simulink model "Assignment1_2020a"  (R2020a)
settings: Solver=FixedStepAuto  StartTime=0.0  StopTime=30  FixedStep=1e-3  RelTol=1e-3  EnableMultiTasking=on
undefined symbols (not defined in the file): A0, A1, D0, D1, D10, D11, D12, D13, D2, D3, D4, D5, D6, D7, D8, D9, PTA0, PTA1, PTA2, PTB2, PTB23, PTB3, PTB9, PTC16, PTC17, PTC2, PTC3, PTC4, PTD0, PTD1, PTD2, PTD3
libraries: frdmk64flib x23, etargetslib x2, dspstat3 x1
settings Model: ExtModeTrigDuration=5  Creator=raymo  LastModifiedBy=raymo
settings OptimizationCC: EnhancedBackFolding=on  PassReuseOutputArgsAs=Individual arguments  ZeroExternalMemoryAtStartup=off  ZeroInternalMemoryAtStartup=off  MaxStackSize=64  OptimizeBlockOrder=speed  DifferentSizesBufferReuse=on  OptimizationCustomize=off  EfficientTunableParamExpr=on
settings DebuggingCC: ParameterTunabilityLossMsg=error
settings HardwareCC: ProdBitPerPointer=32  ProdBitPerSizeT=32  ProdBitPerPtrDiffT=32  ProdLargestAtomicInteger=Long  ProdLargestAtomicFloat=Double  ProdWordSize=32  ProdHWDeviceType=ARM Compatible->ARM Cortex
settings SFSimCC: MATLABDynamicMemAlloc=off
settings RTWCC: SystemTargetFile=ert.tlc  HardwareBoard=NXP FRDM-K64F  TemplateMakefile=ert_default_tmf  Toolchain=GNU Tools for ARM Embedded Processors
settings CodeAppCC: ForceParamTrailComments=on  IgnoreCustomStorageClasses=off  OperatorAnnotations=on  SimulinkDataObjDesc=on  SFDataObjDesc=on  InsertBlockDesc=on

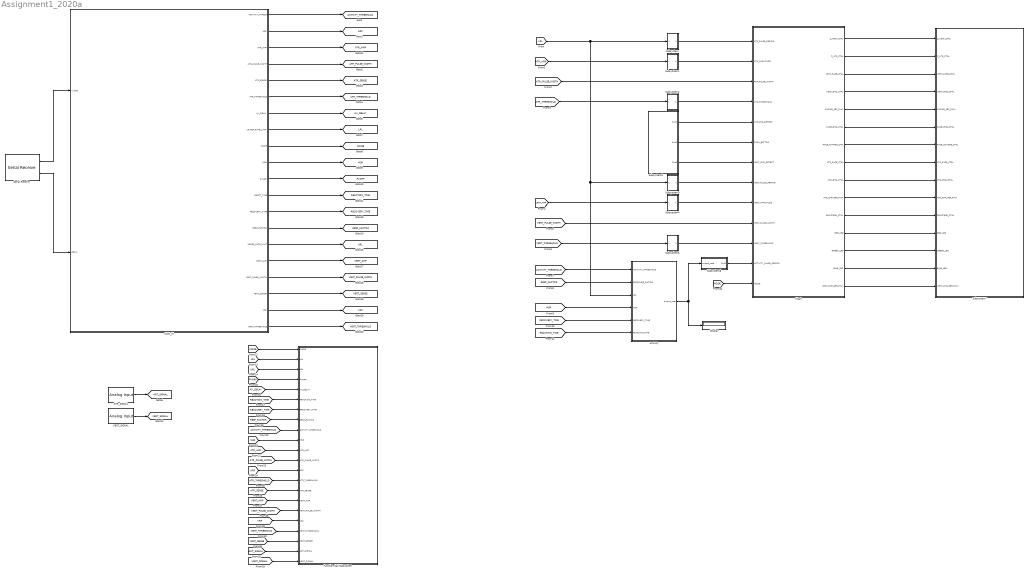
== system Assignment1_2020a ==
  ATR_SIGNAL : frdmk64flib/Analog Input  Whichpin=PTB2 (A0)  SampleTime=-1
  Activity : Subsystem
  COM_IN : Stateflow chart  TreatAsAtomicUnit=on
  Chart : Stateflow chart  TreatAsAtomicUnit=on
      settings: PortSchema="{\"entries\":[{\"content\":{\"sides\":[{\"content\":{\"connectorIds\":[\"In1\",\"In2\",\"In3\",\"In4\",\"In5\",\"In6\",\"In9\",\"In7\",\"In8\",\"In10\",\"In11\",\"In12\",\"In13\"]},\"type\":\"ConnectorPlacement.EquallySpacedRectSide\",\"uuid\":\"1d074b9c-7cc8-4198-85a6-5618993573f0\"},{\"content\":{\"connectorIds\":[\"Out1\",\"Out2\",\"Out3\",\"Out4\",\"Out5\",\"Out6\",\"Out7\",\"Out8\",\"Out9\",\"Out10\",\"Out11\",\"Out12\",\"Out13\",\"Out14\",\"Out15\"],\"side\":\"RIGHT\"},\"type\":\"ConnectorPlacement.EquallySpacedRectSide\",\"uuid\":\"14c2042e-8be8-4cb1-bcfb-7c1019a33e21\"},{\"content\":{\"connectorIds\":[],\"side\":\"TOP\"},\"type\":\"ConnectorPlacement.EquallySpacedRectSide\",\"uuid\":\"e4fcd7b9-cecf-490a-a51f-afb907c3ace7\"}]},\"type\":\"ConnectorPlacement.EquallySpacedConnector\",\"uuid\":\"e4f7c1e4-ab35-4f24-879f-75d9e4e0e882\"}],\"packageUris\":[\"http://schema.mathworks.com/mf0/Connector/19700101\"],\"version\":\"1.0\"}"
  Display : Display
  Function-Call Subsystem : Subsystem  TreatAsAtomicUnit=on
  Serial Receive : frdmk64flib/Serial Receive  SCIModule=0  Baudrate=uint32(9600)  Parity=None  StopBits=1  HardwareFlowControl=None  ByteOrder=LittleEndian  DataType=uint8  DataLength=11  BlockingMode=off  OutputStatus=on  SampleTime=-1
  Subsystem : Subsystem
  Subsystem1 : Subsystem
  Subsystem2 : Subsystem
  Subsystem3 : Subsystem
  Subsystem4 : Subsystem
  Subsystem5 : Subsystem
  Subsystem6 : Subsystem
  Subsystem7 : Subsystem
  Subsystem8 : Subsystem
  VENT_SIGNAL : frdmk64flib/Analog Input  Whichpin=PTB3 (A1)  SampleTime=-1
  tag scope: ACTIVITY_THRESHOLD=global, ARP=global, ART_SIGNAL=global, ATR_AMP=global, ATR_PULSE_WIDTH=global, ATR_SENSE=global, ATR_THRESHOLD=global, AV_DELAY=global, LRL=global, MODE=global, MSR=global, PVARP=global, REACTION_TIME=global, RECOVERY_TIME=global, RESP_FACTOR=global, URL=global, VENT_AMP=global, VENT_PULSE_WIDTH=global, VENT_SENSE=global, VENT_SIGNAL=global, VENT_THRESHOLD=global, VRP=global
  wires:
  [ATR_PULSE_WIDTH] -> Chart/3(ATR_PULSE_WIDTH)
  Subsystem/1(Out1) -> Chart/1(ATR_PULSE_PERIOD)
  [ATR_AMP] -> Subsystem1/1(In1)
  Subsystem1/1(Out1) -> Chart/2(ATR_AMPLITUDE)
  [ATR_THRESHOLD] -> Subsystem2/1(In1)
  Subsystem2/1(Out1) -> Chart/4(ATR_THRESHOLD)
  Subsystem3/1(Out1) -> Chart/7(VENT_PULSE_PERIOD)
  [LRL] -> Subsystem3/1(In1), Activity/3(LRL), Subsystem/1(In1)
  [VENT_AMP] -> Subsystem4/1(In1)
  Subsystem4/1(Out1) -> Chart/8(VENT_AMPLITUDE)
  [VENT_THRESHOLD] -> Subsystem5/1(In1)
  Subsystem5/1(Out1) -> Chart/11(VENT_THRESHOLD)
  Subsystem6/1(Out1) -> Chart/5(ATR_CMP_DETECT)
  Subsystem6/2(Out2) -> Chart/6(PUSH_BUTTON)
  Subsystem6/3(Out3) -> Chart/9(VENT_CMP_DETECT)
  Chart/1(Z_VENT_CTRL) -> Subsystem7/1(Z_VENT_CTRL)
  Chart/2(Z_ATR_CTRL) -> Subsystem7/2(Z_ATR_CTRL)
  Chart/3(VENT_PACE_CTRL) -> Subsystem7/3(VENT_PACE_CTRL)
  Chart/4(VENT_GND_CTRL) -> Subsystem7/4(VENT_GND_CTRL)
  Chart/5(PACING_REF_PWM) -> Subsystem7/5(PACING_REF_PWM)
  Chart/6(PACE_GND_CTRL) -> Subsystem7/6(PACE_GND_CTRL)
  Chart/7(PACE_CHARGE_CTRL) -> Subsystem7/7(PACE_CHARGE_CTRL)
  Chart/8(ATR_PACE_CTRL) -> Subsystem7/8(ATR_PACE_CTRL)
  Chart/9(ATR_GND_CTRL) -> Subsystem7/9(ATR_GND_CTRL)
  Chart/10(ATR_CMP_REF_PWM) -> Subsystem7/10(ATR_CMP_REF_PWM)
  Chart/11(FRONTEND_CTRL) -> Subsystem7/11(FRONTEND_CTRL)
  Chart/12(RED_LED) -> Subsystem7/12(RED_LED)
  Chart/13(GREEN_LED) -> Subsystem7/13(GREEN_LED)
  Chart/15(VENT_CMP_REF_PWM) -> Subsystem7/15(VENT_CMP_REF_PWM)
  Activity/1(output_rate) -> Display/1, Subsystem8/1(output_rate)
  Subsystem8/1(Out1) -> Chart/12(ACTIVITY_PULSE_PERIOD)
  Chart/14(BLUE_LED) -> Subsystem7/14(BLUE_LED)
  Serial Receive/1 -> COM_IN/1(rxdata)
  Serial Receive/2 -> COM_IN/2(status)
  COM_IN/1(ACTIVITY_THRESH) -> [ACTIVITY_THRESHOLD]
  COM_IN/2(ARP) -> [ARP]
  COM_IN/3(ATR_AMP) -> [ATR_AMP]
  COM_IN/4(ATR_PULSE_WIDTH) -> [ATR_PULSE_WIDTH]
  COM_IN/5(ATR_SENSE) -> [ATR_SENSE]
  COM_IN/8(LOWER_RATE_LIMIT) -> [LRL]
  COM_IN/6(ATR_THRESHOLD) -> [ATR_THRESHOLD]
  COM_IN/7(AV_DELAY) -> [AV_DELAY]
  COM_IN/9(MODE) -> [MODE]
  COM_IN/10(MSR) -> [MSR]
  COM_IN/11(PVARP) -> [PVARP]
  COM_IN/13(RECOVERY_TIME) -> [RECOVERY_TIME]
  COM_IN/12(REACT_TIME) -> [REACTION_TIME]
  COM_IN/16(VENT_AMP) -> [VENT_AMP]
  COM_IN/14(RESP_FACTOR) -> [RESP_FACTOR]
  COM_IN/15(UPPER_RATE_LIMIT) -> [URL]
  COM_IN/18(VENT_SENSE) -> [VENT_SENSE]
  COM_IN/17(VENT_PULSE_WIDTH) -> [VENT_PULSE_WIDTH]
  COM_IN/20(VENT_THRESHOLD) -> [VENT_THRESHOLD]
  COM_IN/19(VRP) -> [VRP]
  [ACTIVITY_THRESHOLD] -> Activity/1(ACTIVITY_THRESHOLD)
  [RESP_FACTOR] -> Activity/2(RESPONSE_FACTOR)
  [MSR] -> Activity/4(MSR)
  [RECOVERY_TIME] -> Activity/5(RECOVERY_TIME)
  [REACTION_TIME] -> Activity/6(REACTION_TIME)
  [MODE] -> Function-Call Subsystem/1(MODE)
  [LRL] -> Function-Call Subsystem/2(LRL)
  [URL] -> Function-Call Subsystem/3(URL)
  [AV_DELAY] -> Function-Call Subsystem/5(AV_DELAY)
  [PVARP] -> Function-Call Subsystem/4(PVARP)
  [REACTION_TIME] -> Function-Call Subsystem/6(REACTION_TIME)
  [RESP_FACTOR] -> Function-Call Subsystem/8(RESP_FACTOR)
  [RECOVERY_TIME] -> Function-Call Subsystem/7(RECOVERY_TIME)
  [ACTIVITY_THRESHOLD] -> Function-Call Subsystem/9(ACTIVITY_TRESHOLD)
  [ATR_AMP] -> Function-Call Subsystem/11(ATR_AMP)
  [MSR] -> Function-Call Subsystem/10(MSR)
  [ATR_PULSE_WIDTH] -> Function-Call Subsystem/12(ATR_PULSE_WIDTH)
  [ATR_THRESHOLD] -> Function-Call Subsystem/14(ATR_THRESHOLD)
  [ARP] -> Function-Call Subsystem/13(ARP)
  [ATR_SENSE] -> Function-Call Subsystem/15(ATR_SENSE)
  [VENT_PULSE_WIDTH] -> Function-Call Subsystem/17(VENT_PULSE_WIDTH)
  [VENT_AMP] -> Function-Call Subsystem/16(VENT_AMP)
  [VRP] -> Function-Call Subsystem/18(VRP)
  [VENT_SIGNAL] -> Function-Call Subsystem/22(VENT_SIGNAL)
  [VENT_THRESHOLD] -> Function-Call Subsystem/19(VENT_THRESHOLD)
  [ART_SIGNAL] -> Function-Call Subsystem/21(ART_SIGNAL)
  [VENT_SENSE] -> Function-Call Subsystem/20(VENT_SENSE)
  ATR_SIGNAL/1 -> [ART_SIGNAL]
  VENT_SIGNAL/1 -> [VENT_SIGNAL]
  [VENT_PULSE_WIDTH] -> Chart/10(VENT_PULSE_WIDTH)
  [MODE] -> Chart/13(MODE)

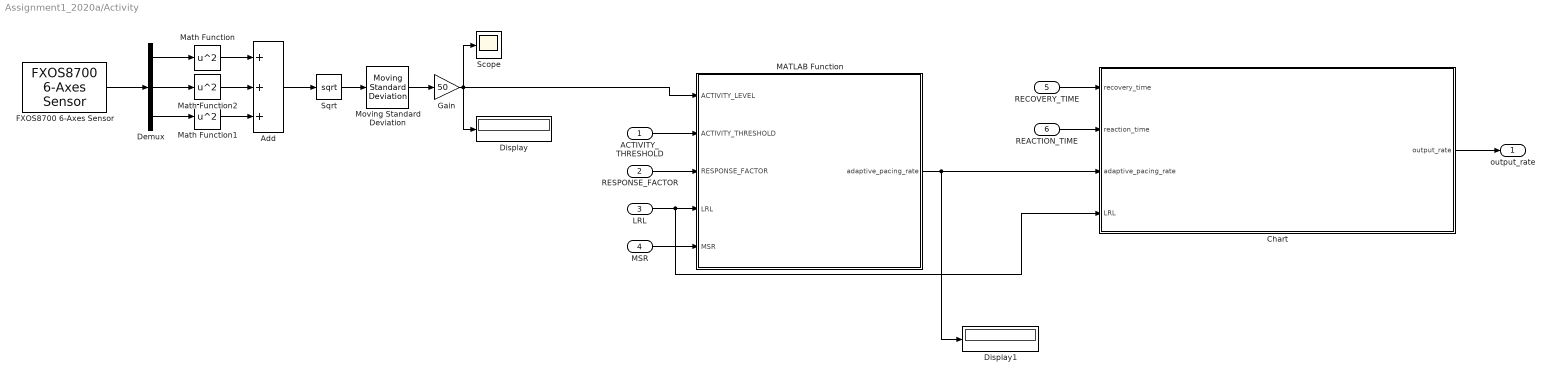
== system Assignment1_2020a/Activity ==
  ACTIVITY_THRESHOLD : Inport
  RESPONSE_FACTOR : Inport  Port=2
  LRL : Inport  Port=3
  MSR : Inport  Port=4
  RECOVERY_TIME : Inport  Port=5
  REACTION_TIME : Inport  Port=6
  Add : Sum  Inputs=+++
  Chart : Stateflow chart  TreatAsAtomicUnit=on
  Demux : Demux  Outputs=3
  Display : Display
  Display1 : Display
  FXOS8700 6-Axes Sensor : frdmk64flib/FXOS8700 6-Axes Sensor  Activesensor=Accelerometer only  ODR=800Hz  HybridODR=400Hz  Accelfullrange=-4g to +4g  SampleTime=-1
  Gain : Gain  Gain=50
  MATLAB Function : MATLAB Function  TreatAsAtomicUnit=on
  Math Function : Math  Operator=square  SaturateOnIntegerOverflow=on
  Math Function1 : Math  Operator=square  SaturateOnIntegerOverflow=on
  Math Function2 : Math  Operator=square  SaturateOnIntegerOverflow=on
  Moving Standard Deviation : dspstat3/Moving Standard Deviation  Method=Sliding window  ForgettingFactorPort=off  SpecifyWindowLength=on  WindowLength=4  ForgettingFactor=0.9  SimulateUsing=Interpreted execution
      settings: SourceProductBaseCode=DS
  Scope : Scope
  Sqrt : Sqrt  SaturateOnIntegerOverflow=on
  output_rate : Outport
  wires:
  FXOS8700 6-Axes Sensor/1 -> Demux/1
  Demux/3 -> Math Function1/1
  Demux/2 -> Math Function2/1
  Demux/1 -> Math Function/1
  Math Function/1 -> Add/1
  Math Function2/1 -> Add/2
  Math Function1/1 -> Add/3
  Add/1 -> Sqrt/1
  Sqrt/1 -> Moving Standard Deviation/1
  Moving Standard Deviation/1 -> Gain/1
  Gain/1 -> Display/1, MATLAB Function/1(ACTIVITY_LEVEL), Scope/1
  ACTIVITY_THRESHOLD/1 -> MATLAB Function/2(ACTIVITY_THRESHOLD)
  RESPONSE_FACTOR/1 -> MATLAB Function/3(RESPONSE_FACTOR)
  LRL/1 -> Chart/4(LRL), MATLAB Function/4(LRL)
  MSR/1 -> MATLAB Function/5(MSR)
  MATLAB Function/1(adaptive_pacing_rate) -> Display1/1, Chart/3(adaptive_pacing_rate)
  RECOVERY_TIME/1 -> Chart/1(recovery_time)
  REACTION_TIME/1 -> Chart/2(reaction_time)
  Chart/1(output_rate) -> output_rate/1

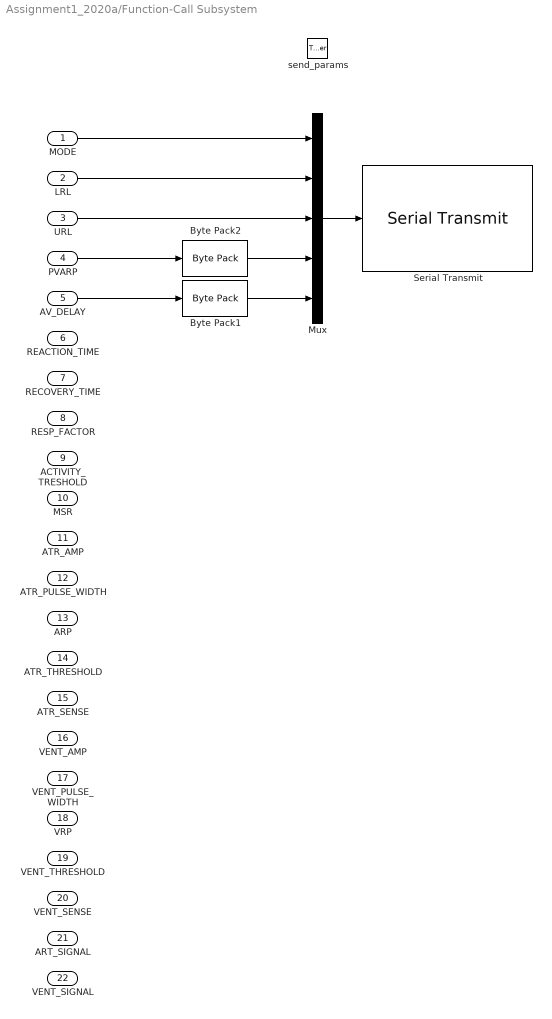
== system Assignment1_2020a/Function-Call Subsystem ==
  MODE : Inport  OutDataTypeStr=uint8
  LRL : Inport  Port=2  OutDataTypeStr=uint8
  URL : Inport  Port=3  OutDataTypeStr=uint8
  PVARP : Inport  Port=4  OutDataTypeStr=single
  AV_DELAY : Inport  Port=5  OutDataTypeStr=uint16
  REACTION_TIME : Inport  Port=6  OutDataTypeStr=uint16
  RECOVERY_TIME : Inport  Port=7  OutDataTypeStr=uint8
  RESP_FACTOR : Inport  Port=8  OutDataTypeStr=uint8
  ACTIVITY_TRESHOLD : Inport  Port=9  OutDataTypeStr=uint8
  MSR : Inport  Port=10  OutDataTypeStr=single
  ATR_AMP : Inport  Port=11  OutDataTypeStr=uint16
  ATR_PULSE_WIDTH : Inport  Port=12  OutDataTypeStr=uint16
  ARP : Inport  Port=13  OutDataTypeStr=uint8
  ATR_THRESHOLD : Inport  Port=14  OutDataTypeStr=uint8
  ATR_SENSE : Inport  Port=15  OutDataTypeStr=uint8
  VENT_AMP : Inport  Port=16  OutDataTypeStr=single
  VENT_PULSE_WIDTH : Inport  Port=17  OutDataTypeStr=uint16
  VRP : Inport  Port=18  OutDataTypeStr=uint16
  VENT_THRESHOLD : Inport  Port=19  OutDataTypeStr=uint8
  VENT_SENSE : Inport  Port=20  OutDataTypeStr=uint8
  ART_SIGNAL : Inport  Port=21  OutDataTypeStr=uint8
  VENT_SIGNAL : Inport  Port=22  OutDataTypeStr=single
  send_params : TriggerPort  TriggerType=function-call  IsSimulinkFunction=on  FunctionName=send_params  VariantControl=Variant
  Byte Pack1 : etargetslib/Byte Pack  datatypes={'uint16'}  byteAlign=1
  Byte Pack2 : etargetslib/Byte Pack  datatypes={'single'}  byteAlign=1
  Mux : Mux  Inputs=5
  Serial Transmit : frdmk64flib/Serial Transmit  SCIModule=0  Baudrate=uint32(9600)  Parity=None  StopBits=1  HardwareFlowControl=None  ByteOrder=LittleEndian  BlockingMode=on  OutputStatus=off
  wires:
  LRL/1 -> Mux/2
  AV_DELAY/1 -> Byte Pack1/1
  Mux/1 -> Serial Transmit/1
  PVARP/1 -> Byte Pack2/1
  Byte Pack1/1 -> Mux/5
  URL/1 -> Mux/3
  MODE/1 -> Mux/1
  Byte Pack2/1 -> Mux/4

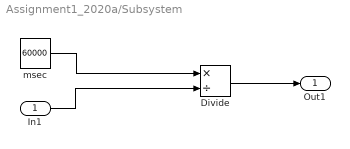
== system Assignment1_2020a/Subsystem ==
  In1 : Inport
  Divide : Product  Inputs=*/
  msec : Constant  Value=60000
  Out1 : Outport
  wires:
  Divide/1 -> Out1/1
  msec/1 -> Divide/1
  In1/1 -> Divide/2

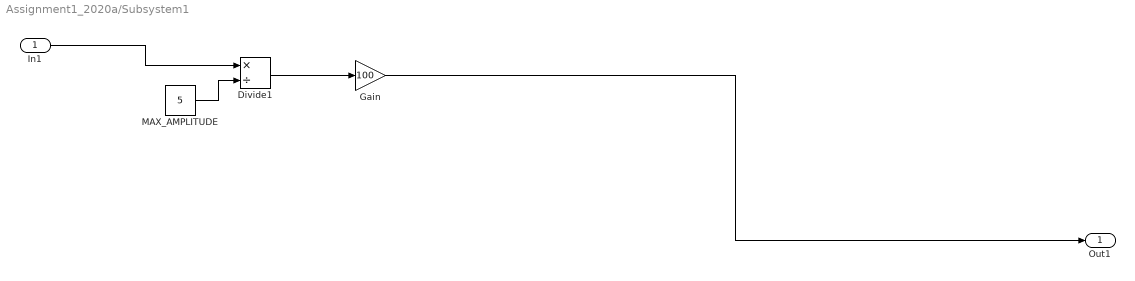
== system Assignment1_2020a/Subsystem1 ==
  In1 : Inport
  Divide1 : Product  Inputs=*/
  Gain : Gain  Gain=100
  MAX_AMPLITUDE : Constant  Value=5
  Out1 : Outport
  wires:
  Gain/1 -> Out1/1
  MAX_AMPLITUDE/1 -> Divide1/2
  In1/1 -> Divide1/1
  Divide1/1 -> Gain/1

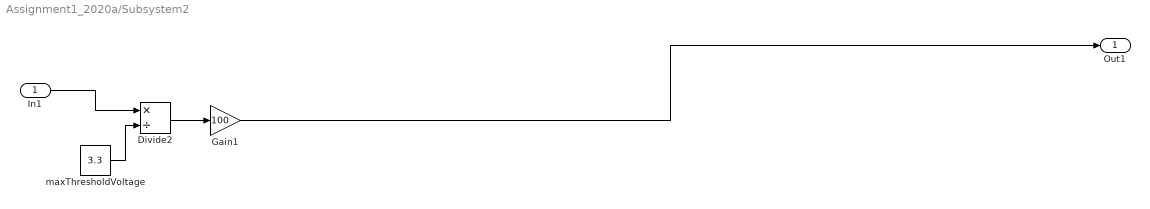
== system Assignment1_2020a/Subsystem2 ==
  In1 : Inport
  Divide2 : Product  Inputs=*/
  Gain1 : Gain  Gain=100
  maxThresholdVoltage : Constant  Value=3.3
  Out1 : Outport
  wires:
  Divide2/1 -> Gain1/1
  maxThresholdVoltage/1 -> Divide2/2
  In1/1 -> Divide2/1
  Gain1/1 -> Out1/1

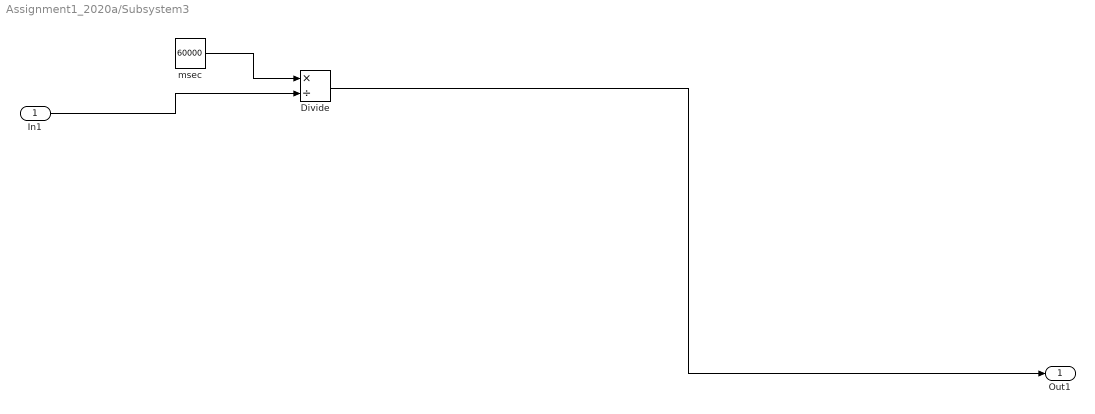
== system Assignment1_2020a/Subsystem3 ==
  In1 : Inport
  Divide : Product  Inputs=*/
  msec : Constant  Value=60000
  Out1 : Outport
  wires:
  Divide/1 -> Out1/1
  msec/1 -> Divide/1
  In1/1 -> Divide/2

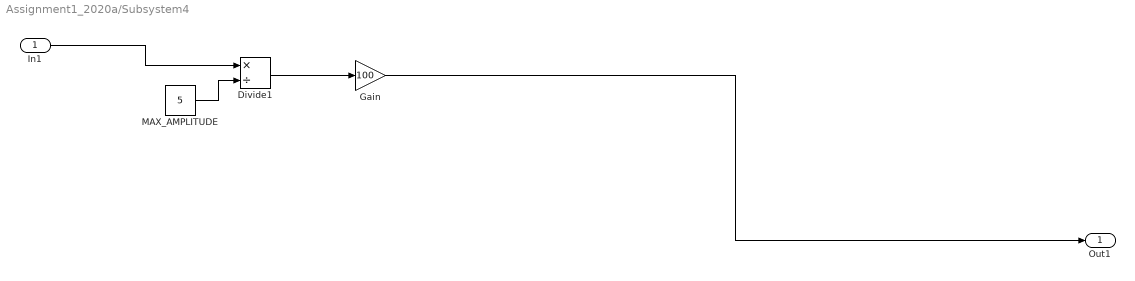
== system Assignment1_2020a/Subsystem4 ==
  In1 : Inport
  Divide1 : Product  Inputs=*/
  Gain : Gain  Gain=100
  MAX_AMPLITUDE : Constant  Value=5
  Out1 : Outport
  wires:
  Gain/1 -> Out1/1
  MAX_AMPLITUDE/1 -> Divide1/2
  In1/1 -> Divide1/1
  Divide1/1 -> Gain/1

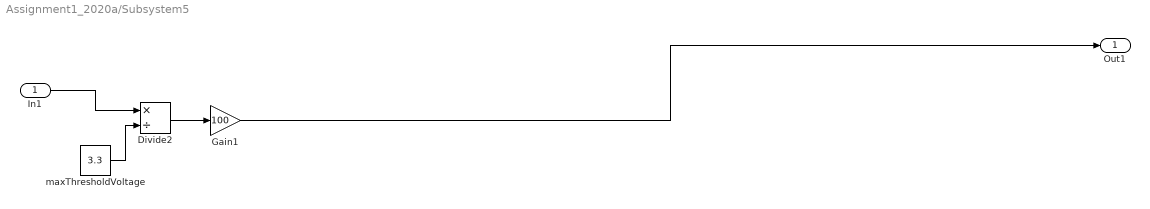
== system Assignment1_2020a/Subsystem5 ==
  In1 : Inport
  Divide2 : Product  Inputs=*/
  Gain1 : Gain  Gain=100
  maxThresholdVoltage : Constant  Value=3.3
  Out1 : Outport
  wires:
  Divide2/1 -> Gain1/1
  maxThresholdVoltage/1 -> Divide2/2
  In1/1 -> Divide2/1
  Gain1/1 -> Out1/1

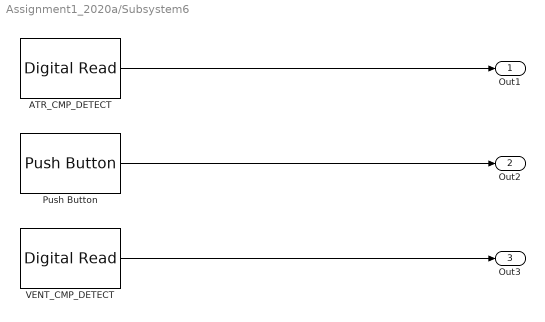
== system Assignment1_2020a/Subsystem6 ==
  ATR_CMP_DETECT : frdmk64flib/Digital Read  Whichpin=PTC16 (D0)  SampleTime=-1
  Push Button : frdmk64flib/Push Button  Whichswitch=SW2  SampleTime1=-1
  VENT_CMP_DETECT : frdmk64flib/Digital Read  Whichpin=PTC17 (D1)  SampleTime=-1
  Out1 : Outport
  Out2 : Outport  Port=2
  Out3 : Outport  Port=3
  wires:
  VENT_CMP_DETECT/1 -> Out3/1
  ATR_CMP_DETECT/1 -> Out1/1
  Push Button/1 -> Out2/1

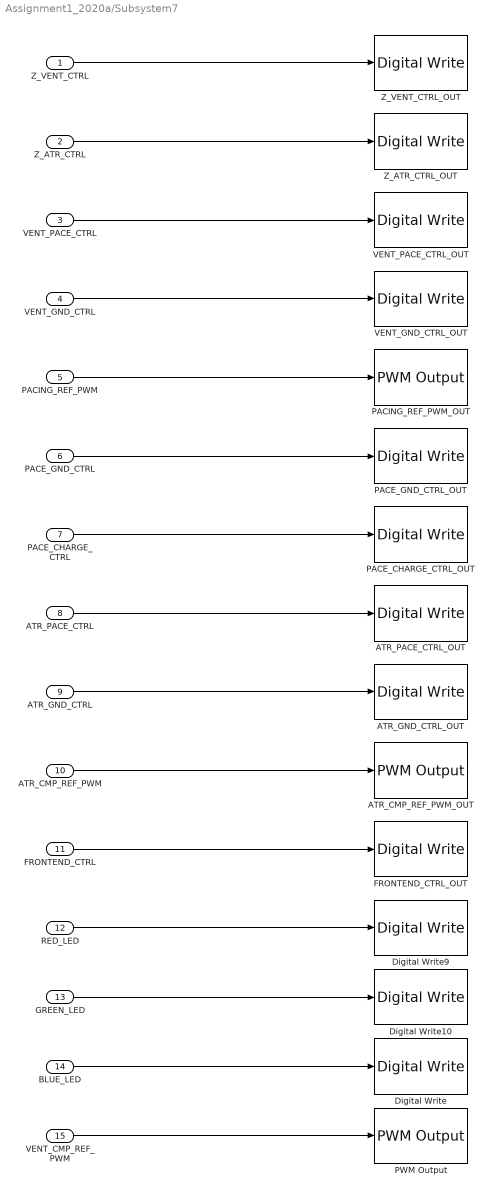
== system Assignment1_2020a/Subsystem7 ==
  Z_VENT_CTRL : Inport
  Z_ATR_CTRL : Inport  Port=2
  VENT_PACE_CTRL : Inport  Port=3
  VENT_GND_CTRL : Inport  Port=4
  PACING_REF_PWM : Inport  Port=5
  PACE_GND_CTRL : Inport  Port=6
  PACE_CHARGE_CTRL : Inport  Port=7
  ATR_PACE_CTRL : Inport  Port=8
  ATR_GND_CTRL : Inport  Port=9
  ATR_CMP_REF_PWM : Inport  Port=10
  FRONTEND_CTRL : Inport  Port=11
  RED_LED : Inport  Port=12
  GREEN_LED : Inport  Port=13
  BLUE_LED : Inport  Port=14
  VENT_CMP_REF_PWM : Inport  Port=15
  ATR_CMP_REF_PWM_OUT : frdmk64flib/PWM Output  Whichpin=PTC2 (D6)  InitialFrequency=2000  InitialDutyCycle=50
  ATR_GND_CTRL_OUT : frdmk64flib/Digital Write  Whichpin=PTD2 (D11)
  ATR_PACE_CTRL_OUT : frdmk64flib/Digital Write  Whichpin=PTA0 (D8)
  Digital Write : frdmk64flib/Digital Write  Whichpin=BLUE_LED
  Digital Write10 : frdmk64flib/Digital Write  Whichpin=GREEN_LED
  Digital Write9 : frdmk64flib/Digital Write  Whichpin=RED_LED
  FRONTEND_CTRL_OUT : frdmk64flib/Digital Write  Whichpin=PTD1 (D13)
  PACE_CHARGE_CTRL_OUT : frdmk64flib/Digital Write  Whichpin=PTB9 (D2)
  PACE_GND_CTRL_OUT : frdmk64flib/Digital Write  Whichpin=PTD0 (D10)
  PACING_REF_PWM_OUT : frdmk64flib/PWM Output  Whichpin=PTA2 (D5)  InitialFrequency=2000  InitialDutyCycle=50
  PWM Output : frdmk64flib/PWM Output  Whichpin=PTA1 (D3)  InitialFrequency=2000  InitialDutyCycle=0
  VENT_GND_CTRL_OUT : frdmk64flib/Digital Write  Whichpin=PTD3 (D12)
  VENT_PACE_CTRL_OUT : frdmk64flib/Digital Write  Whichpin=PTC4 (D9)
  Z_ATR_CTRL_OUT : frdmk64flib/Digital Write  Whichpin=PTB23 (D4)
  Z_VENT_CTRL_OUT : frdmk64flib/Digital Write  Whichpin=PTC3 (D7)
  wires:
  ATR_PACE_CTRL/1 -> ATR_PACE_CTRL_OUT/1
  PACE_GND_CTRL/1 -> PACE_GND_CTRL_OUT/1
  Z_VENT_CTRL/1 -> Z_VENT_CTRL_OUT/1
  PACE_CHARGE_CTRL/1 -> PACE_CHARGE_CTRL_OUT/1
  GREEN_LED/1 -> Digital Write10/1
  ATR_CMP_REF_PWM/1 -> ATR_CMP_REF_PWM_OUT/1
  RED_LED/1 -> Digital Write9/1
  ATR_GND_CTRL/1 -> ATR_GND_CTRL_OUT/1
  FRONTEND_CTRL/1 -> FRONTEND_CTRL_OUT/1
  VENT_GND_CTRL/1 -> VENT_GND_CTRL_OUT/1
  PACING_REF_PWM/1 -> PACING_REF_PWM_OUT/1
  VENT_PACE_CTRL/1 -> VENT_PACE_CTRL_OUT/1
  Z_ATR_CTRL/1 -> Z_ATR_CTRL_OUT/1
  VENT_CMP_REF_PWM/1 -> PWM Output/1
  BLUE_LED/1 -> Digital Write/1

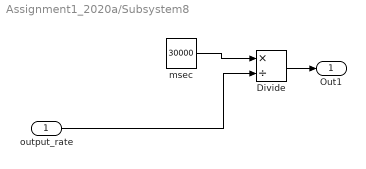
== system Assignment1_2020a/Subsystem8 ==
  output_rate : Inport
  Divide : Product  Inputs=*/
  msec : Constant  Value=30000
  Out1 : Outport
  wires:
  output_rate/1 -> Divide/2
  msec/1 -> Divide/1
  Divide/1 -> Out1/1

== stateflow chart Assignment1_2020a/Activity/Chart ==
  state IDLE
    entry:
    output_rate = LRL;
  state INIT
    entry:
    %The slope of the time response curves
    step_up = abs((adaptive_pacing_rate - output_rate)/reaction_time);
    step_down = abs((adaptive_pacing_rate - output_rate)/recovery_time);
  state STEP_DOWN
    entry:
    output_rate = output_rate - step_down;
  state STEP_UP
    entry:
    output_rate = output_rate + step_up;
  (default) -> IDLE
  IDLE -> INIT
  INIT -> STEP_DOWN [order 2] : [output_rate > adaptive_pacing_rate]
  INIT -> STEP_UP [order 1] : [output_rate < adaptive_pacing_rate]
  STEP_UP -> INIT : [after(1000,msec)]
  STEP_DOWN -> INIT : [after(1000,msec)]
  data: recovery_time input; reaction_time input; adaptive_pacing_rate input; LRL input; step_down local; step_up local; output_rate output

== matlab function Assignment1_2020a/Activity/MATLAB Function ==
  data: ACTIVITY_LEVEL input; adaptive_pacing_rate output; ACTIVITY_THRESHOLD input; RESPONSE_FACTOR input; LRL input; MSR input
function adaptive_pacing_rate = fcn(ACTIVITY_LEVEL, ACTIVITY_THRESHOLD, RESPONSE_FACTOR, LRL , MSR)
    if ACTIVITY_LEVEL <= ACTIVITY_THRESHOLD
        adaptive_pacing_rate = LRL; 
    else
        slope = 2.5*RESPONSE_FACTOR;
        b = LRL - (slope*ACTIVITY_THRESHOLD);
        linear_rate_response = (slope*ACTIVITY_LEVEL) + b;
        if(linear_rate_response >= MSR)
           adaptive_pacing_rate = MSR;
        else
            adaptive_pacing_rate = linear_rate_response;
        end
    end
end

== stateflow chart Assignment1_2020a/Chart ==
  state IDLE
  state AOO
    state ChargeDishcharge
      entry:
      %C22
      ATR_PACE_CTRL = 0;
      VENT_PACE_CTRL = 0;
      PACING_REF_PWM = ATR_AMPLITUDE;
      PACE_CHARGE_CTRL = 1;
      %C21
      PACE_GND_CTRL = 1;
      VENT_PACE_CTRL = 0;
      Z_ATR_CTRL = 0;
      Z_VENT_CTRL = 0;
      ATR_GND_CTRL = 1;
      VENT_GND_CTRL = 0;
      %LED
      RED_LED = 0;
      GREEN_LED = 0;
      BLUE_LED = 0;
    state AVpacing
      entry:
      PACE_CHARGE_CTRL = 0;
      PACE_GND_CTRL = 1;
      ATR_PACE_CTRL = 1;
      ATR_GND_CTRL = 0;
      Z_ATR_CTRL = 0;
      Z_VENT_CTRL = 0;
      VENT_GND_CTRL = 0;
      VENT_PACE_CTRL = 0;
      PACING_REF_PWM = ATR_AMPLITUDE;
    (default) -> AOO.ChargeDishcharge
    AOO.AVpacing -> AOO.ChargeDishcharge : [after(ATR_PULSE_WIDTH, msec)]
    AOO.ChargeDishcharge -> AOO.AVpacing : [after(ATR_PULSE_PERIOD-ATR_PULSE_WIDTH, msec)]
  state AAI
    state Idle
      entry:
      %Set threshold
      ATR_CMP_REF_PWM = ATR_THRESHOLD;
      FRONTEND_CTRL = 1;
      RED_LED = 1;
      GREEN_LED = 0;
      BLUE_LED = 0;
    state AVpacing
      entry:
      PACE_CHARGE_CTRL = 0;
      PACE_GND_CTRL = 1;
      ATR_PACE_CTRL = 1;
      ATR_GND_CTRL = 0;
      Z_ATR_CTRL = 0;
      Z_VENT_CTRL = 0;
      VENT_GND_CTRL = 0;
      VENT_PACE_CTRL = 0;
      PACING_REF_PWM = ATR_AMPLITUDE;
    state ChargeDischarge
      entry:
      %C22
      ATR_PACE_CTRL = 0;
      VENT_PACE_CTRL = 0;
      PACING_REF_PWM = ATR_AMPLITUDE;
      PACE_CHARGE_CTRL = 1;
      %C21
      PACE_GND_CTRL = 1;
      VENT_PACE_CTRL = 0;
      Z_ATR_CTRL = 0;
      Z_VENT_CTRL = 0;
      ATR_GND_CTRL = 1;
      VENT_GND_CTRL = 0;
    (default) -> AAI.Idle
    AAI.Idle -> AAI.ChargeDischarge
    AAI.ChargeDischarge -> AAI.ChargeDischarge [order 1] : after(5,msec)[ATR_CMP_DETECT == 1]
    AAI.ChargeDischarge -> AAI.AVpacing [order 2] : [after(ATR_PULSE_PERIOD-ATR_PULSE_WIDTH,msec)]
    AAI.AVpacing -> AAI.ChargeDischarge : [after(ATR_PULSE_WIDTH, msec)]
  state VOO
    state Pacing
      entry:
      PACE_CHARGE_CTRL=0;
      PACE_GND_CTRL=1;
      ATR_PACE_CTRL=0;
      ATR_GND_CTRL=0;
      Z_ATR_CTRL=0;
      Z_VENT_CTRL=0;
      VENT_GND_CTRL=0;
      VENT_PACE_CTRL=1;
    state Charging
      entry:
      ATR_PACE_CTRL=0;
      VENT_PACE_CTRL=0;
      PACING_REF_PWM=VENT_AMPLITUDE;
      PACE_CHARGE_CTRL=1;
      RED_LED = 0;
      GREEN_LED = 1;
      BLUE_LED = 0;
    state Discharging
      entry:
      PACE_GND_CTRL=1;
      VENT_PACE_CTRL=0;
      Z_ATR_CTRL=0;
      Z_VENT_CTRL=0;
      ATR_PACE_CTRL=0;
      ATR_GND_CTRL=0;
      VENT_GND_CTRL=1;
    (default) -> VOO.Charging
    VOO.Charging -> VOO.Pacing : [after(VENT_PULSE_PERIOD,msec)]
    VOO.Discharging -> VOO.Charging
    VOO.Pacing -> VOO.Discharging : [after(VENT_PULSE_WIDTH,msec)]
  state VVI
    state Initialization
      entry:
      FRONTEND_CTRL = 1;
      VENT_CMP_REF_PWM = VENT_THRESHOLD;
      RED_LED = 1;
      GREEN_LED = 1;
      BLUE_LED = 0;
    state Pacing
      entry:
      PACE_CHARGE_CTRL=0;
      PACE_GND_CTRL=1;
      ATR_PACE_CTRL=0;
      ATR_GND_CTRL=0;
      Z_ATR_CTRL=0;
      Z_VENT_CTRL=0;
      VENT_GND_CTRL=0;
      VENT_PACE_CTRL=1;
    state Charging
      entry:
      ATR_PACE_CTRL=0;
      VENT_PACE_CTRL=0;
      PACING_REF_PWM=VENT_AMPLITUDE;
      PACE_CHARGE_CTRL=1;
    state Discharging
      entry:
      PACE_GND_CTRL=1;
      VENT_PACE_CTRL=0;
      Z_ATR_CTRL=0;
      Z_VENT_CTRL=0;
      ATR_PACE_CTRL=0;
      ATR_GND_CTRL=0;
      VENT_GND_CTRL=1;
    (default) -> Initialization
    VVI.Charging -> VVI.Charging [order 1] : after(5,msec)[VENT_CMP_DETECT == 1]
    Initialization -> VVI.Charging
    VVI.Charging -> VVI.Pacing [order 2] : [after(VENT_PULSE_PERIOD-VENT_PULSE_WIDTH,msec)]
    VVI.Discharging -> VVI.Charging
    VVI.Pacing -> VVI.Discharging : [after(VENT_PULSE_WIDTH,msec)]
  state AOOR
    state ChargeDishcharge
      entry:
      %C22
      ATR_PACE_CTRL = 0;
      VENT_PACE_CTRL = 0;
      PACING_REF_PWM = ATR_AMPLITUDE;
      PACE_CHARGE_CTRL = 1;
      %C21
      PACE_GND_CTRL = 1;
      VENT_PACE_CTRL = 0;
      Z_ATR_CTRL = 0;
      Z_VENT_CTRL = 0;
      ATR_GND_CTRL = 1;
      VENT_GND_CTRL = 0;
      %LED
      RED_LED = 0;
      GREEN_LED = 0;
      BLUE_LED = 1;
    state AVpacing
      entry:
      PACE_CHARGE_CTRL = 0;
      PACE_GND_CTRL = 1;
      ATR_PACE_CTRL = 1;
      ATR_GND_CTRL = 0;
      Z_ATR_CTRL = 0;
      Z_VENT_CTRL = 0;
      VENT_GND_CTRL = 0;
      VENT_PACE_CTRL = 0;
      PACING_REF_PWM = ATR_AMPLITUDE;
    (default) -> AOOR.ChargeDishcharge
    AOOR.AVpacing -> AOOR.ChargeDishcharge : [after(ATR_PULSE_WIDTH, msec)]
    AOOR.ChargeDishcharge -> AOOR.AVpacing : [after(ACTIVITY_PULSE_PERIOD-ATR_PULSE_WIDTH, msec)]
  state AAIR
    state Idle
      entry:
      %Set threshold
      ATR_CMP_REF_PWM = ATR_THRESHOLD;
      FRONTEND_CTRL = 1;
      RED_LED = 1;
      GREEN_LED = 0;
      BLUE_LED = 0;
    state AVpacing
      entry:
      PACE_CHARGE_CTRL = 0;
      PACE_GND_CTRL = 1;
      ATR_PACE_CTRL = 1;
      ATR_GND_CTRL = 0;
      Z_ATR_CTRL = 0;
      Z_VENT_CTRL = 0;
      VENT_GND_CTRL = 0;
      VENT_PACE_CTRL = 0;
      PACING_REF_PWM = ATR_AMPLITUDE;
    state ChargeDischarge
      entry:
      %C22
      ATR_PACE_CTRL = 0;
      VENT_PACE_CTRL = 0;
      PACING_REF_PWM = ATR_AMPLITUDE;
      PACE_CHARGE_CTRL = 1;
      %C21
      PACE_GND_CTRL = 1;
      VENT_PACE_CTRL = 0;
      Z_ATR_CTRL = 0;
      Z_VENT_CTRL = 0;
      ATR_GND_CTRL = 1;
      VENT_GND_CTRL = 0;
    (default) -> AAIR.Idle
    AAIR.Idle -> AAIR.ChargeDischarge
    AAIR.ChargeDischarge -> AAIR.ChargeDischarge [order 1] : after(5,msec)[ATR_CMP_DETECT == 1]
    AAIR.ChargeDischarge -> AAIR.AVpacing [order 2] : [after(ATIVITY_PULSE_PERIOD-ATR_PULSE_WIDTH,msec)]
    AAIR.AVpacing -> AAIR.ChargeDischarge : [after(ATR_PULSE_WIDTH, msec)]
  state VOOR
    state Pacing
      entry:
      PACE_CHARGE_CTRL=0;
      PACE_GND_CTRL=1;
      ATR_PACE_CTRL=0;
      ATR_GND_CTRL=0;
      Z_ATR_CTRL=0;
      Z_VENT_CTRL=0;
      VENT_GND_CTRL=0;
      VENT_PACE_CTRL=1;
    state Charging
      entry:
      ATR_PACE_CTRL=0;
      VENT_PACE_CTRL=0;
      PACING_REF_PWM=VENT_AMPLITUDE;
      PACE_CHARGE_CTRL=1;
      RED_LED = 1;
      GREEN_LED = 0;
      BLUE_LED = 1;
    state Discharging
      entry:
      PACE_GND_CTRL=1;
      VENT_PACE_CTRL=0;
      Z_ATR_CTRL=0;
      Z_VENT_CTRL=0;
      ATR_PACE_CTRL=0;
      ATR_GND_CTRL=0;
      VENT_GND_CTRL=1;
    (default) -> VOOR.Charging
    VOOR.Charging -> VOOR.Pacing : [after(ACTIVITY_PULSE_PERIOD,msec)]
    VOOR.Discharging -> VOOR.Charging
    VOOR.Pacing -> VOOR.Discharging : [after(VENT_PULSE_WIDTH,msec)]
  state VVIR
    state Pacing
      entry:
      PACE_CHARGE_CTRL=0;
      PACE_GND_CTRL=1;
      ATR_PACE_CTRL=0;
      ATR_GND_CTRL=0;
      Z_ATR_CTRL=0;
      Z_VENT_CTRL=0;
      VENT_GND_CTRL=0;
      VENT_PACE_CTRL=1;
    state Charging
      entry:
      ATR_PACE_CTRL=0;
      VENT_PACE_CTRL=0;
      PACING_REF_PWM=VENT_AMPLITUDE;
      PACE_CHARGE_CTRL=1;
      RED_LED = 0;
      GREEN_LED = 1;
      BLUE_LED = 0;
    state Discharging
      entry:
      PACE_GND_CTRL=1;
      VENT_PACE_CTRL=0;
      Z_ATR_CTRL=0;
      Z_VENT_CTRL=0;
      ATR_PACE_CTRL=0;
      ATR_GND_CTRL=0;
      VENT_GND_CTRL=1;
    (default) -> VVIR.Charging
    VVIR.Charging -> VVIR.Pacing : [after(ACTIVITY_PULSE_PERIOD,msec)]
    VVIR.Discharging -> VVIR.Charging
    VVIR.Pacing -> VVIR.Discharging : [after(VENT_PULSE_WIDTH,msec)]
  (default) -> IDLE
  IDLE -> AOO [order 1] : [MODE == 1]
  AOO -> IDLE : [MODE ~= 1]
  IDLE -> AAI [order 2] : [MODE == 2]
  AAI -> IDLE : [MODE ~= 2]
  IDLE -> VOO [order 3] : [MODE == 3]
  VOO -> IDLE : [MODE ~= 3]
  IDLE -> VVI [order 4] : [MODE == 4]
  VVI -> IDLE : [MODE ~= 4]
  IDLE -> AOOR [order 5] : [MODE == 5]
  AOOR -> IDLE : [MODE ~= 5]
  IDLE -> AAIR [order 8] : [MODE == 6]
  AAIR -> IDLE : [MODE ~= 6]
  IDLE -> VOOR [order 6] : [MODE == 7]
  VOOR -> IDLE : [MODE ~= 7]
  IDLE -> VVIR [order 7] : [MODE == 8]
  VVIR -> IDLE : [MODE ~= 8]
  data: ATR_PULSE_PERIOD input; ATR_AMPLITUDE input; ATR_PULSE_WIDTH input; ATR_THRESHOLD input; ATR_CMP_DETECT input; Z_VENT_CTRL output; Z_ATR_CTRL output; VENT_PACE_CTRL output; VENT_GND_CTRL output; PACING_REF_PWM output; PACE_GND_CTRL output; PACE_CHARGE_CTRL output; ATR_PACE_CTRL output; ATR_GND_CTRL output; ATR_CMP_REF_PWM output; FRONTEND_CTRL output; PUSH_BUTTON input; RED_LED output; GREEN_LED output; BLUE_LED output; VENT_PULSE_PERIOD input; VENT_CMP_REF_PWM output; VENT_AMPLITUDE input; VENT_CMP_DETECT input; VENT_PULSE_WIDTH input; VENT_THRESHOLD input; ACTIVITY_PULSE_PERIOD input; MODE input

== stateflow chart Assignment1_2020a/COM_IN ==
  settings: executeAtInitialization=1
  state SET_PARAM
    entry:
    MODE = typecast(rxdata(3:4), 'uint16');
    LOWER_RATE_LIMIT = typecast(rxdata(5:6), 'uint16');
    UPPER_RATE_LIMIT = typecast(rxdata(7:8), 'uint16');
    PVARP = typecast(rxdata(9:10), 'uint16');
    AV_DELAY = typecast(rxdata(11:12), 'uint16');
    REACT_TIME = typecast(rxdata(13:14), 'uint16');
    RESP_FACTOR = typecast(rxdata(15:16), 'uint16');
    ACTIVITY_THRESH = typecast(rxdata(17:24), 'double');
    RECOVERY_TIME = typecast(rxdata(25:26), 'uint16');
    MSR = typecast(rxdata(27:28), 'uint16');
    %ATR
    ATR_AMP = typecast(rxdata(29:36), 'double');
    ATR_PULSE_WIDTH = typecast(rxdata(37:38), 'uint16');
    ARP = typecast(rxdata(39:40), 'uint16');
    ATR_THRESHOLD = typecast(rxdata(41:48), 'double');
    ATR_SENSE = typecast(rxdata(49:56), 'double');
    %VENT
    VENT_AMP = typecast(rxdata(57:64), 'double');
    VENT_PULSE_WIDTH = typecast(rxdata(65:66), 'uint16');
    VRP = typecast(rxdata(67:68), 'uint16');
    VENT_THRESHOLD = typecast(rxdata(69:76), 'double');
    VENT_SENSE = typecast(rxdata(77:84), 'double');
  state INITIAL
    % Set the init values of parameters
    entry:
    MODE = 0;
    LOWER_RATE_LIMIT = 60;
    UPPER_RATE_LIMIT = 180;
    PVARP = 250;
    AV_DELAY = 150;
    REACT_TIME = 10;
    RESP_FACTOR = 8;
    ACTIVITY_THRESH = 0.2;
    RECOVERY_TIME = 20;
    MSR =180;
    %ATR
    ATR_AMP = 5;
    ATR_PULSE_WIDTH = 10;
    ARP = 0;
    ATR_THRESHOLD = 1.98;
    ATR_SENSE = 0;
    %VENT
    VENT_AMP = 5;
    VENT_PULSE_WIDTH = 10;
    VRP = 0;
    VENT_THRESHOLD = 1.6;
    VENT_SENSE = 0;
  state STANDBY
    %Waiting for COM
  state ECHO_PARAM
    entry:
    send_params();
  SET_PARAM -> STANDBY
  (junction 10) -> SET_PARAM [order 2] : [rxdata(2) == hex2dec('55')]
  (default) -> INITIAL
  (junction 6) -> STANDBY [order 2]
  INITIAL -> STANDBY
  STANDBY -> (junction 6) : [status == 0]
  (junction 6) -> (junction 10) [order 1] : [rxdata(1) == hex2dec('16')]
  (junction 10) -> ECHO_PARAM [order 1] : [rxdata(2) == hex2dec('22')]
  ECHO_PARAM -> STANDBY
  data: rxdata input uint8; status input uint8; ACTIVITY_THRESH output; ARP output; ATR_AMP output; ATR_PULSE_WIDTH output; ATR_SENSE output; ATR_THRESHOLD output; AV_DELAY output; LOWER_RATE_LIMIT output; MODE output; MSR output; PVARP output; REACT_TIME output; RECOVERY_TIME output; RESP_FACTOR output; UPPER_RATE_LIMIT output; VENT_AMP output; VENT_PULSE_WIDTH output; VENT_SENSE output; VRP output; VENT_THRESHOLD output
